simulink model "Mooventure2016_Rev5"  (Simulink 7.7)
settings: Solver=FixedStepDiscrete  StartTime=0.0  StopTime=10  RelTol=1e-3
PreLoadFcn:
  | try, eval([bdroot '_setup']); catch, eval('model_setup', ''); end
InitFcn:
  | try, eval([bdroot '_setup']); catch, eval('model_setup', ''); end
undefined symbols (not defined in the file): ECM, H1, motohawk_build_version, motohawk_trunc_name, motohawk_vardec_config_group, motohawk_vardec_path, xD
libraries: MotoHawk_lib x976, motohawk_control_primitives_lib x41, simulink x27, motohawk_annotations_lib x3
(part 12 of 16)

== system Mooventure2016_Rev5/Foreground/Control/Faults/Accesories/Blend Valves ==
  In1 : Inport
  Abs : Abs
  Abs1 : Abs
  Add1 : Sum  Inputs=+-
  Add2 : Sum  Inputs=+-
  Bus Selector1 : BusSelector  OutputSignals=Analog_Inputs.Coolant.Heater_Core_Blend_Position
  Bus Selector2 : BusSelector  OutputSignals=Analog_Inputs.Coolant.Radiator_Blend_Position
  Bus Selector3 : BusSelector  OutputSignals=Analog_Inputs.Coolant.Radiator_Blend_Position
  Bus Selector4 : BusSelector  OutputSignals=Analog_Inputs.Coolant.Radiator_Blend_Position
  Bus Selector5 : BusSelector  OutputSignals=Analog_Inputs.Coolant.Heater_Core_Blend_Position
  Bus Selector6 : BusSelector  OutputSignals=Analog_Inputs.Coolant.Heater_Core_Blend_Position
  Logical Operator : Logic  AllPortsSameDT=off  OutDataTypeStr=boolean
  Logical Operator1 : Logic  AllPortsSameDT=off  OutDataTypeStr=boolean
  Relational Operator{,4,6..7} (4 alike) : RelationalOperator  Operator=>  OutDataTypeStr=boolean
  Relational Operator1 : RelationalOperator  OutDataTypeStr=boolean
  Relational Operator2 : RelationalOperator  OutDataTypeStr=boolean
  Relational Operator3 : RelationalOperator  Operator=<  OutDataTypeStr=boolean
  Relational Operator5 : RelationalOperator  Operator=<  OutDataTypeStr=boolean
  Time Since Enabled (With Input)1 : motohawk_control_primitives_lib/Time Since Enabled (With Input)1  SystemSampleTime=-1  nam='TimeSinceRun1'  samp_time=-1  init=0  upperlim=16000
  Time Since Enabled (With Input)2 : motohawk_control_primitives_lib/Time Since Enabled (With Input)1  SystemSampleTime=-1  nam='TimeSinceRun2'  samp_time=-1  init=0  upperlim=16000
  Unit Delay : UnitDelay  SampleTime=-1
  Unit Delay1 : UnitDelay  SampleTime=-1
  motohawk_calibration : MotoHawk_lib/Calibration & Probing Blocks/motohawk_calibration  nam='Blend_Valve_A_No_Response_Fault'  val=100  storage=Calibration  show_more=off  name_source=Use Parameter  data_type=Inherit from 'Default Value'  read_level=1  write_level=1  ovr_cals=on  view_as=Number  enum_struct={'Disabled', 'Enabled'}  vector_style=Wide Row  use_help_units=off  help=''  units=''  use_header_enum=off  row_header_enum={}  col_header_enum={}  use_min_max=off  min_val=-inf  max_val=inf  use_precision=off  precision=''  gain=1  offset=0  exp=1  use_mototune_group=off  mototune_group=motohawk_vardec_path(gcb)
  motohawk_calibration1 : MotoHawk_lib/Calibration & Probing Blocks/motohawk_calibration  nam='Blend_Valve_Sensor_B_Intermittent_Fault'  val=4  storage=Calibration  show_more=off  name_source=Use Parameter  data_type=Inherit from 'Default Value'  read_level=1  write_level=1  ovr_cals=on  view_as=Number  enum_struct={'Disabled', 'Enabled'}  vector_style=Wide Row  use_help_units=off  help=''  units=''  use_header_enum=off  row_header_enum={}  col_header_enum={}  use_min_max=off  min_val=-inf  max_val=inf  use_precision=off  precision=''  gain=1  offset=0  exp=1  use_mototune_group=off  mototune_group=motohawk_vardec_path(gcb)
  motohawk_calibration2 : MotoHawk_lib/Calibration & Probing Blocks/motohawk_calibration  nam='Blend_Valve_Sensor_A_Intermittent_Fault'  val=4  storage=Calibration  show_more=off  name_source=Use Parameter  data_type=Inherit from 'Default Value'  read_level=1  write_level=1  ovr_cals=on  view_as=Number  enum_struct={'Disabled', 'Enabled'}  vector_style=Wide Row  use_help_units=off  help=''  units=''  use_header_enum=off  row_header_enum={}  col_header_enum={}  use_min_max=off  min_val=-inf  max_val=inf  use_precision=off  precision=''  gain=1  offset=0  exp=1  use_mototune_group=off  mototune_group=motohawk_vardec_path(gcb)
  motohawk_calibration3 : MotoHawk_lib/Calibration & Probing Blocks/motohawk_calibration  nam='Blend_Valve_Sensor_A_Low_Voltage_Fault'  val=5  storage=Calibration  show_more=off  name_source=Use Parameter  data_type=Inherit from 'Default Value'  read_level=1  write_level=1  ovr_cals=on  view_as=Number  enum_struct={'Disabled', 'Enabled'}  vector_style=Wide Row  use_help_units=off  help=''  units=''  use_header_enum=off  row_header_enum={}  col_header_enum={}  use_min_max=off  min_val=-inf  max_val=inf  use_precision=off  precision=''  gain=1  offset=0  exp=1  use_mototune_group=off  mototune_group=motohawk_vardec_path(gcb)
  motohawk_calibration4 : MotoHawk_lib/Calibration & Probing Blocks/motohawk_calibration  nam='Blend_Valve_Sensor_A_High_Voltage_Fault'  val=250  storage=Calibration  show_more=off  name_source=Use Parameter  data_type=Inherit from 'Default Value'  read_level=1  write_level=1  ovr_cals=on  view_as=Number  enum_struct={'Disabled', 'Enabled'}  vector_style=Wide Row  use_help_units=off  help=''  units=''  use_header_enum=off  row_header_enum={}  col_header_enum={}  use_min_max=off  min_val=-inf  max_val=inf  use_precision=off  precision=''  gain=1  offset=0  exp=1  use_mototune_group=off  mototune_group=motohawk_vardec_path(gcb)
  motohawk_calibration5 : MotoHawk_lib/Calibration & Probing Blocks/motohawk_calibration  nam='Blend_Valve_Sensor_B_Low_Voltage_Fault'  val=5  storage=Calibration  show_more=off  name_source=Use Parameter  data_type=Inherit from 'Default Value'  read_level=1  write_level=1  ovr_cals=on  view_as=Number  enum_struct={'Disabled', 'Enabled'}  vector_style=Wide Row  use_help_units=off  help=''  units=''  use_header_enum=off  row_header_enum={}  col_header_enum={}  use_min_max=off  min_val=-inf  max_val=inf  use_precision=off  precision=''  gain=1  offset=0  exp=1  use_mototune_group=off  mototune_group=motohawk_vardec_path(gcb)
  motohawk_calibration6 : MotoHawk_lib/Calibration & Probing Blocks/motohawk_calibration  nam='Blend_Valve_Sensor_B_High_Voltage_Fault'  val=250  storage=Calibration  show_more=off  name_source=Use Parameter  data_type=Inherit from 'Default Value'  read_level=1  write_level=1  ovr_cals=on  view_as=Number  enum_struct={'Disabled', 'Enabled'}  vector_style=Wide Row  use_help_units=off  help=''  units=''  use_header_enum=off  row_header_enum={}  col_header_enum={}  use_min_max=off  min_val=-inf  max_val=inf  use_precision=off  precision=''  gain=1  offset=0  exp=1  use_mototune_group=off  mototune_group=motohawk_vardec_path(gcb)
  motohawk_calibration7 : MotoHawk_lib/Calibration & Probing Blocks/motohawk_calibration  nam='Blend_Valve_B_No_Response_Fault'  val=100  storage=Calibration  show_more=off  name_source=Use Parameter  data_type=Inherit from 'Default Value'  read_level=1  write_level=1  ovr_cals=on  view_as=Number  enum_struct={'Disabled', 'Enabled'}  vector_style=Wide Row  use_help_units=off  help=''  units=''  use_header_enum=off  row_header_enum={}  col_header_enum={}  use_min_max=off  min_val=-inf  max_val=inf  use_precision=off  precision=''  gain=1  offset=0  exp=1  use_mototune_group=off  mototune_group=motohawk_vardec_path(gcb)
  motohawk_fault_def1 : MotoHawk_lib/Fault Management Blocks/motohawk_fault_def  nam='Blend_Valve_Sensor_B_Intermittent'  mode=Enabled  id=['B1B43']  x=9  y=10  input_suspected=on  indeterminate=off  increment_xy=on  downsample_count=1  ovr_cals=on  ovr_actions=on  show_actions=on  action1_name=''  action1_cond=(None)  action2_name=''  action2_cond=(None)  action3_name=''  action3_cond=(None)  action4_name=''  action4_cond=(None)
  motohawk_fault_def2 : MotoHawk_lib/Fault Management Blocks/motohawk_fault_def  nam='Blend_Valve_Sensor_B_Low_Voltage'  mode=Enabled  id=['B1B44']  x=9  y=10  input_suspected=on  indeterminate=off  increment_xy=on  downsample_count=1  ovr_cals=on  ovr_actions=on  show_actions=on  action1_name=''  action1_cond=(None)  action2_name=''  action2_cond=(None)  action3_name=''  action3_cond=(None)  action4_name=''  action4_cond=(None)
  motohawk_fault_def3 : MotoHawk_lib/Fault Management Blocks/motohawk_fault_def  nam='Blend_Valve_Sensor_A_Intermittent'  mode=Enabled  id=['B1B40']  x=9  y=10  input_suspected=on  indeterminate=off  increment_xy=on  downsample_count=1  ovr_cals=on  ovr_actions=on  show_actions=on  action1_name=''  action1_cond=(None)  action2_name=''  action2_cond=(None)  action3_name=''  action3_cond=(None)  action4_name=''  action4_cond=(None)
  motohawk_fault_def4 : MotoHawk_lib/Fault Management Blocks/motohawk_fault_def  nam='Blend_Valve_Sensor_A_Low_Voltage'  mode=Enabled  id=['B1B41']  x=9  y=10  input_suspected=on  indeterminate=off  increment_xy=on  downsample_count=1  ovr_cals=on  ovr_actions=on  show_actions=on  action1_name=''  action1_cond=(None)  action2_name=''  action2_cond=(None)  action3_name=''  action3_cond=(None)  action4_name=''  action4_cond=(None)
  motohawk_fault_def5 : MotoHawk_lib/Fault Management Blocks/motohawk_fault_def  nam='Blend_Valve_Sensor_A_High_Voltage'  mode=Enabled  id=['B1B42']  x=9  y=10  input_suspected=on  indeterminate=off  increment_xy=on  downsample_count=1  ovr_cals=on  ovr_actions=on  show_actions=on  action1_name=''  action1_cond=(None)  action2_name=''  action2_cond=(None)  action3_name=''  action3_cond=(None)  action4_name=''  action4_cond=(None)
  motohawk_fault_def6 : MotoHawk_lib/Fault Management Blocks/motohawk_fault_def  nam='Blend_Valve_Sensor_B_High_Voltage'  mode=Enabled  id=['B1B45']  x=9  y=10  input_suspected=on  indeterminate=off  increment_xy=on  downsample_count=1  ovr_cals=on  ovr_actions=on  show_actions=on  action1_name=''  action1_cond=(None)  action2_name=''  action2_cond=(None)  action3_name=''  action3_cond=(None)  action4_name=''  action4_cond=(None)
  motohawk_fault_def7 : MotoHawk_lib/Fault Management Blocks/motohawk_fault_def  nam='Blend_Valve_A_No_Response'  mode=Enabled  id=['B1B46']  x=9  y=10  input_suspected=on  indeterminate=off  increment_xy=on  downsample_count=1  ovr_cals=on  ovr_actions=on  show_actions=on  action1_name=''  action1_cond=(None)  action2_name=''  action2_cond=(None)  action3_name=''  action3_cond=(None)  action4_name=''  action4_cond=(None)
  motohawk_fault_def8 : MotoHawk_lib/Fault Management Blocks/motohawk_fault_def  nam='Blend_Valve_B_No_Response'  mode=Enabled  id=['B1B47']  x=9  y=10  input_suspected=on  indeterminate=off  increment_xy=on  downsample_count=1  ovr_cals=on  ovr_actions=on  show_actions=on  action1_name=''  action1_cond=(None)  action2_name=''  action2_cond=(None)  action3_name=''  action3_cond=(None)  action4_name=''  action4_cond=(None)
  wires:
  Bus Selector2/1 -> Add1/1, Unit Delay/1  "<Radiator_Blend_Position>"
  Unit Delay/1 -> Add1/2
  Add1/1 -> Abs/1
  Abs/1 -> Relational Operator2/1
  Relational Operator2/1 -> motohawk_fault_def3/1
  motohawk_calibration2/1 -> Relational Operator2/2
  motohawk_calibration3/1 -> Relational Operator3/2
  Relational Operator3/1 -> motohawk_fault_def4/1
  Bus Selector3/1 -> Relational Operator3/1  "<Radiator_Blend_Position>"
  motohawk_calibration4/1 -> Relational Operator4/2
  Relational Operator4/1 -> motohawk_fault_def5/1
  Bus Selector4/1 -> Relational Operator4/1  "<Radiator_Blend_Position>"
  In1/1 -> Bus Selector2/1, Bus Selector3/1, Bus Selector4/1, Bus Selector1/1, Bus Selector5/1, Bus Selector6/1
  Bus Selector1/1 -> Add2/1, Unit Delay1/1  "<Heater_Core_Blend_Position>"
  Unit Delay1/1 -> Add2/2
  Add2/1 -> Abs1/1
  Abs1/1 -> Relational Operator1/1
  Relational Operator1/1 -> motohawk_fault_def1/1
  motohawk_calibration1/1 -> Relational Operator1/2
  motohawk_calibration5/1 -> Relational Operator5/2
  Relational Operator5/1 -> motohawk_fault_def2/1
  Bus Selector5/1 -> Relational Operator5/1  "<Heater_Core_Blend_Position>"
  motohawk_calibration6/1 -> Relational Operator6/2
  Relational Operator6/1 -> motohawk_fault_def6/1
  Bus Selector6/1 -> Relational Operator6/1  "<Heater_Core_Blend_Position>"
  [RadiatorMotor] -> Time Since Enabled (With Input)1/1, Logical Operator/2
  [HeaterMotor] -> Time Since Enabled (With Input)2/1, Logical Operator1/2
  motohawk_calibration/1 -> Relational Operator/2
  Time Since Enabled (With Input)1/1 -> Relational Operator/1
  Time Since Enabled (With Input)2/1 -> Relational Operator7/1
  motohawk_calibration7/1 -> Relational Operator7/2
  Relational Operator/1 -> Logical Operator/1
  Relational Operator7/1 -> Logical Operator1/1
  Logical Operator/1 -> motohawk_fault_def7/1
  Logical Operator1/1 -> motohawk_fault_def8/1

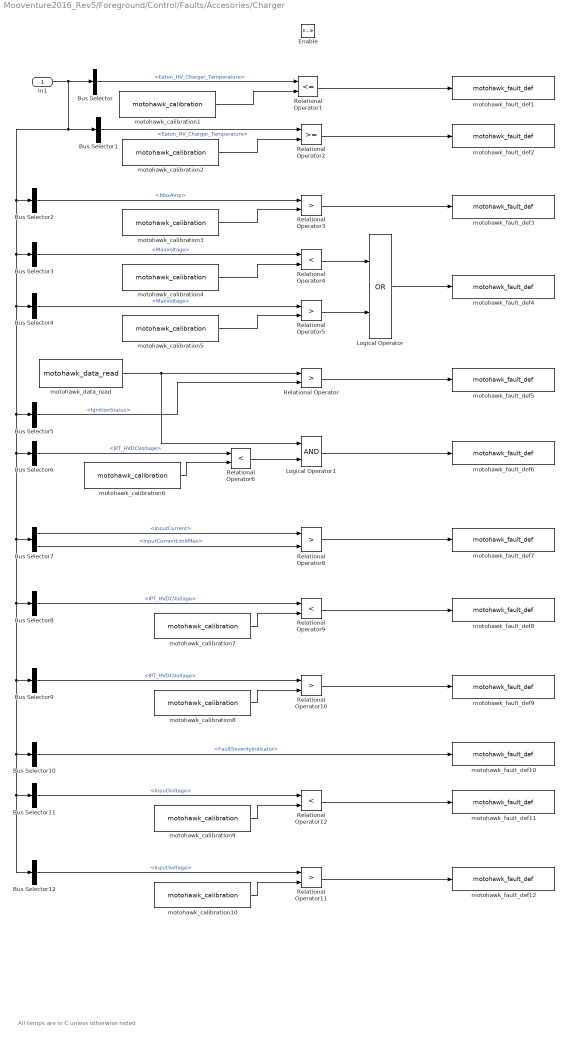
== system Mooventure2016_Rev5/Foreground/Control/Faults/Accesories/Charger ==
  note: All temps are in C unless otherwise noted
  In1 : Inport
  Enable : EnablePort
  Bus Selector : BusSelector  OutputSignals=Eaton_Charger.Eaton_Charger.Eaton_HV_Charger_Temperature
  Bus Selector1 : BusSelector  OutputSignals=Eaton_Charger.Eaton_Charger.Eaton_HV_Charger_Temperature
  Bus Selector10 : BusSelector  OutputSignals=Eaton_Charger.Eaton_Charger.FaultSeverityIndicator
  Bus Selector11 : BusSelector  OutputSignals=Eaton_Charger.Eaton_Charger.InputVoltage
  Bus Selector12 : BusSelector  OutputSignals=Eaton_Charger.Eaton_Charger.InputVoltage
  Bus Selector2 : BusSelector  OutputSignals=ChargerParam.MaxAmp
  Bus Selector3 : BusSelector  OutputSignals=ChargerParam.MaxVoltage
  Bus Selector4 : BusSelector  OutputSignals=ChargerParam.MaxVoltage
  Bus Selector5 : BusSelector  OutputSignals=Eaton_Charger.Eaton_Charger.IgnitionStatus
  Bus Selector6 : BusSelector  OutputSignals=IPT.ID 278 IPT Status 1.IPT_HVDCVoltage
  Bus Selector7 : BusSelector  OutputSignals=Eaton_Charger.Eaton_Charger.InputCurrent,Eaton_Charger.Eaton_Charger.InputCurrentLimitMax
  Bus Selector8 : BusSelector  OutputSignals=IPT.ID 278 IPT Status 1.IPT_HVDCVoltage
  Bus Selector9 : BusSelector  OutputSignals=IPT.ID 278 IPT Status 1.IPT_HVDCVoltage
  Logical Operator : Logic  Operator=OR  AllPortsSameDT=off  OutDataTypeStr=boolean
  Logical Operator1 : Logic  AllPortsSameDT=off  OutDataTypeStr=boolean
  Relational Operator{,3,5,8,10..11} (6 alike) : RelationalOperator  Operator=>  OutDataTypeStr=boolean
  Relational Operator1 : RelationalOperator  Operator=<=  OutDataTypeStr=boolean
  Relational Operator{4,6,9,12} (4 alike) : RelationalOperator  Operator=<  OutDataTypeStr=boolean
  Relational Operator2 : RelationalOperator  OutDataTypeStr=boolean
  motohawk_calibration1 : MotoHawk_lib/Calibration & Probing Blocks/motohawk_calibration  nam='Charger_Derated_Under_Temperature_Fault'  val=-30  storage=Calibration  show_more=off  name_source=Use Parameter  data_type=Inherit from 'Default Value'  read_level=1  write_level=1  ovr_cals=on  view_as=Number  enum_struct={'Disabled', 'Enabled'}  vector_style=Wide Row  use_help_units=off  help=''  units=''  use_header_enum=off  row_header_enum={}  col_header_enum={}  use_min_max=off  min_val=-inf  max_val=inf  use_precision=off  precision=''  gain=1  offset=0  exp=1  use_mototune_group=off  mototune_group=motohawk_vardec_path(gcb)
  motohawk_calibration10 : MotoHawk_lib/Calibration & Probing Blocks/motohawk_calibration  nam='Charger_Line_Votlage_Too_High_Fault'  val=300  storage=Calibration  show_more=off  name_source=Use Parameter  data_type=Inherit from 'Default Value'  read_level=1  write_level=1  ovr_cals=on  view_as=Number  enum_struct={'Disabled', 'Enabled'}  vector_style=Wide Row  use_help_units=off  help=''  units=''  use_header_enum=off  row_header_enum={}  col_header_enum={}  use_min_max=off  min_val=-inf  max_val=inf  use_precision=off  precision=''  gain=1  offset=0  exp=1  use_mototune_group=off  mototune_group=motohawk_vardec_path(gcb)
  motohawk_calibration2 : MotoHawk_lib/Calibration & Probing Blocks/motohawk_calibration  nam='Charger_Derated_Over_Temperature_Fault'  val=60  storage=Calibration  show_more=off  name_source=Use Parameter  data_type=Inherit from 'Default Value'  read_level=1  write_level=1  ovr_cals=on  view_as=Number  enum_struct={'Disabled', 'Enabled'}  vector_style=Wide Row  use_help_units=off  help=''  units=''  use_header_enum=off  row_header_enum={}  col_header_enum={}  use_min_max=off  min_val=-inf  max_val=inf  use_precision=off  precision=''  gain=1  offset=0  exp=1  use_mototune_group=off  mototune_group=motohawk_vardec_path(gcb)
  motohawk_calibration3 : MotoHawk_lib/Calibration & Probing Blocks/motohawk_calibration  nam='Charger_Requested_Current_Too_High_Fault'  val=16  storage=Calibration  show_more=off  name_source=Use Parameter  data_type=Inherit from 'Default Value'  read_level=1  write_level=1  ovr_cals=on  view_as=Number  enum_struct={'Disabled', 'Enabled'}  vector_style=Wide Row  use_help_units=off  help=''  units=''  use_header_enum=off  row_header_enum={}  col_header_enum={}  use_min_max=off  min_val=-inf  max_val=inf  use_precision=off  precision=''  gain=1  offset=0  exp=1  use_mototune_group=off  mototune_group=motohawk_vardec_path(gcb)
  motohawk_calibration4 : MotoHawk_lib/Calibration & Probing Blocks/motohawk_calibration  nam='Charger_Requested_Voltage_Out_of_Bounds_Fault_Lower'  val=298  storage=Calibration  show_more=off  name_source=Use Parameter  data_type=Inherit from 'Default Value'  read_level=1  write_level=1  ovr_cals=on  view_as=Number  enum_struct={'Disabled', 'Enabled'}  vector_style=Wide Row  use_help_units=off  help=''  units=''  use_header_enum=off  row_header_enum={}  col_header_enum={}  use_min_max=off  min_val=-inf  max_val=inf  use_precision=off  precision=''  gain=1  offset=0  exp=1  use_mototune_group=off  mototune_group=motohawk_vardec_path(gcb)
  motohawk_calibration5 : MotoHawk_lib/Calibration & Probing Blocks/motohawk_calibration  nam='Charger_Requested_Voltage_Out_of_Bounds_Fault_Upper'  val=428  storage=Calibration  show_more=off  name_source=Use Parameter  data_type=Inherit from 'Default Value'  read_level=1  write_level=1  ovr_cals=on  view_as=Number  enum_struct={'Disabled', 'Enabled'}  vector_style=Wide Row  use_help_units=off  help=''  units=''  use_header_enum=off  row_header_enum={}  col_header_enum={}  use_min_max=off  min_val=-inf  max_val=inf  use_precision=off  precision=''  gain=1  offset=0  exp=1  use_mototune_group=off  mototune_group=motohawk_vardec_path(gcb)
  motohawk_calibration6 : MotoHawk_lib/Calibration & Probing Blocks/motohawk_calibration  nam='Charger_Requested_But_No_High_Voltage_Fault'  val=50  storage=Calibration  show_more=off  name_source=Use Parameter  data_type=Inherit from 'Default Value'  read_level=1  write_level=1  ovr_cals=on  view_as=Number  enum_struct={'Disabled', 'Enabled'}  vector_style=Wide Row  use_help_units=off  help=''  units=''  use_header_enum=off  row_header_enum={}  col_header_enum={}  use_min_max=off  min_val=-inf  max_val=inf  use_precision=off  precision=''  gain=1  offset=0  exp=1  use_mototune_group=off  mototune_group=motohawk_vardec_path(gcb)
  motohawk_calibration7 : MotoHawk_lib/Calibration & Probing Blocks/motohawk_calibration  nam='Battery_Voltage_Too_Low_Fault'  val=200  storage=Calibration  show_more=off  name_source=Use Parameter  data_type=Inherit from 'Default Value'  read_level=1  write_level=1  ovr_cals=on  view_as=Number  enum_struct={'Disabled', 'Enabled'}  vector_style=Wide Row  use_help_units=off  help=''  units=''  use_header_enum=off  row_header_enum={}  col_header_enum={}  use_min_max=off  min_val=-inf  max_val=inf  use_precision=off  precision=''  gain=1  offset=0  exp=1  use_mototune_group=off  mototune_group=motohawk_vardec_path(gcb)
  motohawk_calibration8 : MotoHawk_lib/Calibration & Probing Blocks/motohawk_calibration  nam='Battery_Voltage_Too_High_Fault'  val=400  storage=Calibration  show_more=off  name_source=Use Parameter  data_type=Inherit from 'Default Value'  read_level=1  write_level=1  ovr_cals=on  view_as=Number  enum_struct={'Disabled', 'Enabled'}  vector_style=Wide Row  use_help_units=off  help=''  units=''  use_header_enum=off  row_header_enum={}  col_header_enum={}  use_min_max=off  min_val=-inf  max_val=inf  use_precision=off  precision=''  gain=1  offset=0  exp=1  use_mototune_group=off  mototune_group=motohawk_vardec_path(gcb)
  motohawk_calibration9 : MotoHawk_lib/Calibration & Probing Blocks/motohawk_calibration  nam='Charger_Line_Voltage_Too_Low_Fault'  val=100  storage=Calibration  show_more=off  name_source=Use Parameter  data_type=Inherit from 'Default Value'  read_level=1  write_level=1  ovr_cals=on  view_as=Number  enum_struct={'Disabled', 'Enabled'}  vector_style=Wide Row  use_help_units=off  help=''  units=''  use_header_enum=off  row_header_enum={}  col_header_enum={}  use_min_max=off  min_val=-inf  max_val=inf  use_precision=off  precision=''  gain=1  offset=0  exp=1  use_mototune_group=off  mototune_group=motohawk_vardec_path(gcb)
  motohawk_data_read : MotoHawk_lib/Data Storage Blocks/motohawk_data_read  source=Lookup By Name  structure=Scalar  operation=Read scalar from location by index  sz_vec=4  sz_row=2  sz_col=3  typ=boolean  nam='ChargeEnable'  checkNull=on  struct_inst_name='MyData'  struct_nam='MyStruct'
  motohawk_fault_def1 : MotoHawk_lib/Fault Management Blocks/motohawk_fault_def  nam='Charger_Derated_Under_Temperature'  mode=Enabled  id=['B1A10']  x=9  y=10  input_suspected=on  indeterminate=off  increment_xy=on  downsample_count=1  ovr_cals=on  ovr_actions=on  show_actions=on  action1_name='Temperature_Flash'  action1_cond=(None)  action2_name=''  action2_cond=(None)  action3_name=''  action3_cond=(None)  action4_name=''  action4_cond=(None)
  motohawk_fault_def10 : MotoHawk_lib/Fault Management Blocks/motohawk_fault_def  nam='Charger_Internal_Fault'  mode=Enabled  id=['B1A32']  x=9  y=10  input_suspected=on  indeterminate=off  increment_xy=on  downsample_count=1  ovr_cals=on  ovr_actions=on  show_actions=on  action1_name='HV_Light'  action1_cond=Active  action2_name=''  action2_cond=(None)  action3_name=''  action3_cond=(None)  action4_name=''  action4_cond=(None)
  motohawk_fault_def11 : MotoHawk_lib/Fault Management Blocks/motohawk_fault_def  nam='Charger_Line_Voltage_Too_Low'  mode=Enabled  id=['B1A33']  x=9  y=10  input_suspected=on  indeterminate=off  increment_xy=on  downsample_count=1  ovr_cals=on  ovr_actions=on  show_actions=on  action1_name='Wrench_Light'  action1_cond=Active  action2_name=''  action2_cond=(None)  action3_name=''  action3_cond=(None)  action4_name=''  action4_cond=(None)
  motohawk_fault_def12 : MotoHawk_lib/Fault Management Blocks/motohawk_fault_def  nam='Charger_Line_Votlage_Too_High'  mode=Enabled  id=['B1A34']  x=9  y=10  input_suspected=on  indeterminate=off  increment_xy=on  downsample_count=1  ovr_cals=on  ovr_actions=on  show_actions=on  action1_name='Wrench_Light'  action1_cond=Active  action2_name=''  action2_cond=(None)  action3_name=''  action3_cond=(None)  action4_name=''  action4_cond=(None)
  motohawk_fault_def2 : MotoHawk_lib/Fault Management Blocks/motohawk_fault_def  nam='Charger_Derated_Over_Temperature'  mode=Enabled  id=['B1A11']  x=9  y=10  input_suspected=on  indeterminate=off  increment_xy=on  downsample_count=1  ovr_cals=on  ovr_actions=on  show_actions=on  action1_name='Temperature_Solid'  action1_cond=Active  action2_name='Cooling_Max'  action2_cond=(None)  action3_name=''  action3_cond=(None)  action4_name=''  action4_cond=(None)
  motohawk_fault_def3 : MotoHawk_lib/Fault Management Blocks/motohawk_fault_def  nam='Charger_Requested_Current_Too_High'  mode=Enabled  id=['B1A20']  x=9  y=10  input_suspected=on  indeterminate=off  increment_xy=on  downsample_count=1  ovr_cals=on  ovr_actions=on  show_actions=on  action1_name='HV_Light'  action1_cond=Active  action2_name=''  action2_cond=(None)  action3_name=''  action3_cond=(None)  action4_name=''  action4_cond=(None)
  motohawk_fault_def4 : MotoHawk_lib/Fault Management Blocks/motohawk_fault_def  nam='Charger_Requested_Voltage_Out_of_Bounds'  mode=Enabled  id=['B1A21']  x=9  y=10  input_suspected=on  indeterminate=off  increment_xy=on  downsample_count=1  ovr_cals=on  ovr_actions=on  show_actions=on  action1_name='HV_Light'  action1_cond=Active  action2_name=''  action2_cond=(None)  action3_name=''  action3_cond=(None)  action4_name=''  action4_cond=(None)
  motohawk_fault_def5 : MotoHawk_lib/Fault Management Blocks/motohawk_fault_def  nam='Charger_Requested_But_No_Key_Singal'  mode=Enabled  id=['B1A22']  x=9  y=10  input_suspected=on  indeterminate=off  increment_xy=on  downsample_count=1  ovr_cals=on  ovr_actions=on  show_actions=on  action1_name='Wrench_Light'  action1_cond=Active  action2_name=''  action2_cond=(None)  action3_name=''  action3_cond=(None)  action4_name=''  action4_cond=(None)
  motohawk_fault_def6 : MotoHawk_lib/Fault Management Blocks/motohawk_fault_def  nam='Charger_Requested_But_No_High_Voltage'  mode=Enabled  id=['B1A23']  x=9  y=10  input_suspected=on  indeterminate=off  increment_xy=on  downsample_count=1  ovr_cals=on  ovr_actions=on  show_actions=on  action1_name='HV_Light'  action1_cond=Active  action2_name=''  action2_cond=(None)  action3_name=''  action3_cond=(None)  action4_name=''  action4_cond=(None)
  motohawk_fault_def7 : MotoHawk_lib/Fault Management Blocks/motohawk_fault_def  nam='Charger_Amperage_Draw_Greater_Then_Supply'  mode=Enabled  id=['B1A24']  x=9  y=10  input_suspected=on  indeterminate=off  increment_xy=on  downsample_count=1  ovr_cals=on  ovr_actions=on  show_actions=on  action1_name='HV_Light'  action1_cond=Active  action2_name=''  action2_cond=(None)  action3_name=''  action3_cond=(None)  action4_name=''  action4_cond=(None)
  motohawk_fault_def8 : MotoHawk_lib/Fault Management Blocks/motohawk_fault_def  nam='Battery_Voltage_Too_Low'  mode=Enabled  id=['B1A30']  x=9  y=10  input_suspected=on  indeterminate=off  increment_xy=on  downsample_count=1  ovr_cals=on  ovr_actions=on  show_actions=on  action1_name='HV_Light'  action1_cond=Active  action2_name=''  action2_cond=(None)  action3_name=''  action3_cond=(None)  action4_name=''  action4_cond=(None)
  motohawk_fault_def9 : MotoHawk_lib/Fault Management Blocks/motohawk_fault_def  nam='Battery_Voltage_Too_High'  mode=Enabled  id=['B1A31']  x=9  y=10  input_suspected=on  indeterminate=off  increment_xy=on  downsample_count=1  ovr_cals=on  ovr_actions=on  show_actions=on  action1_name='HV_Light'  action1_cond=Active  action2_name=''  action2_cond=(None)  action3_name=''  action3_cond=(None)  action4_name=''  action4_cond=(None)
  wires:
  In1/1 -> Bus Selector/1, Bus Selector1/1, Bus Selector2/1, Bus Selector5/1, Bus Selector6/1, Bus Selector7/1, Bus Selector8/1, Bus Selector9/1, Bus Selector10/1, Bus Selector11/1, Bus Selector12/1, Bus Selector4/1, Bus Selector3/1
  motohawk_calibration1/1 -> Relational Operator1/2
  Relational Operator1/1 -> motohawk_fault_def1/1
  Bus Selector/1 -> Relational Operator1/1  "<Eaton_HV_Charger_Temperature>"
  motohawk_calibration2/1 -> Relational Operator2/2
  Relational Operator2/1 -> motohawk_fault_def2/1
  Bus Selector1/1 -> Relational Operator2/1  "<Eaton_HV_Charger_Temperature>"
  motohawk_calibration3/1 -> Relational Operator3/2
  Relational Operator3/1 -> motohawk_fault_def3/1
  motohawk_calibration4/1 -> Relational Operator4/2
  motohawk_calibration5/1 -> Relational Operator5/2
  Relational Operator4/1 -> Logical Operator/1
  Relational Operator5/1 -> Logical Operator/2
  Logical Operator/1 -> motohawk_fault_def4/1
  Bus Selector5/1 -> Relational Operator/2  "<IgnitionStatus>"
  Relational Operator/1 -> motohawk_fault_def5/1
  motohawk_calibration6/1 -> Relational Operator6/2
  Bus Selector6/1 -> Relational Operator6/1  "<IPT_HVDCVoltage>"
  Relational Operator6/1 -> Logical Operator1/2
  Logical Operator1/1 -> motohawk_fault_def6/1
  Bus Selector7/1 -> Relational Operator8/1  "<InputCurrent>"
  Bus Selector7/2 -> Relational Operator8/2  "<InputCurrentLimitMax>"
  Relational Operator8/1 -> motohawk_fault_def7/1
  motohawk_calibration7/1 -> Relational Operator9/2
  Bus Selector8/1 -> Relational Operator9/1  "<IPT_HVDCVoltage>"
  Relational Operator9/1 -> motohawk_fault_def8/1
  motohawk_calibration8/1 -> Relational Operator10/2
  Bus Selector9/1 -> Relational Operator10/1  "<IPT_HVDCVoltage>"
  Relational Operator10/1 -> motohawk_fault_def9/1
  Bus Selector10/1 -> motohawk_fault_def10/1  "<FaultSeverityIndicator>"
  motohawk_calibration9/1 -> Relational Operator12/2
  Bus Selector11/1 -> Relational Operator12/1  "<InputVoltage>"
  Relational Operator12/1 -> motohawk_fault_def11/1
  motohawk_calibration10/1 -> Relational Operator11/2
  Bus Selector12/1 -> Relational Operator11/1  "<InputVoltage>"
  Relational Operator11/1 -> motohawk_fault_def12/1
  Bus Selector2/1 -> Relational Operator3/1  "<MaxAmp>"
  Bus Selector3/1 -> Relational Operator4/1  "<MaxVoltage>"
  Bus Selector4/1 -> Relational Operator5/1  "<MaxVoltage>"
  motohawk_data_read/1 -> Relational Operator/1, Logical Operator1/1

== system Mooventure2016_Rev5/Foreground/Control/Faults/Accesories/DC-DC Converter ==
  In1 : Inport
  Bus Selector : BusSelector  OutputSignals=Analog_Inputs.DCDC
  Relational Operator1 : RelationalOperator  Operator=<  OutDataTypeStr=boolean
  motohawk_calibration1 : MotoHawk_lib/Calibration & Probing Blocks/motohawk_calibration  nam='DCDC_Converter_Not_Running_Fault'  val=200  storage=Calibration  show_more=off  name_source=Use Parameter  data_type=Inherit from 'Default Value'  read_level=1  write_level=1  ovr_cals=on  view_as=Number  enum_struct={'Disabled', 'Enabled'}  vector_style=Wide Row  use_help_units=off  help=''  units=''  use_header_enum=off  row_header_enum={}  col_header_enum={}  use_min_max=off  min_val=-inf  max_val=inf  use_precision=off  precision=''  gain=1  offset=0  exp=1  use_mototune_group=off  mototune_group=motohawk_vardec_path(gcb)
  motohawk_fault_def1 : MotoHawk_lib/Fault Management Blocks/motohawk_fault_def  nam='DCDC_Converter_Not_Running'  mode=Disabled  id=['B1B11']  x=9  y=10  input_suspected=on  indeterminate=off  increment_xy=on  downsample_count=1  ovr_cals=on  ovr_actions=on  show_actions=on  action1_name='Batt_Light'  action1_cond=Active  action2_name=''  action2_cond=(None)  action3_name=''  action3_cond=(None)  action4_name=''  action4_cond=(None)
  wires:
  motohawk_calibration1/1 -> Relational Operator1/2
  Relational Operator1/1 -> motohawk_fault_def1/1
  Bus Selector/1 -> Relational Operator1/1  "<DCDC>"
  In1/1 -> Bus Selector/1

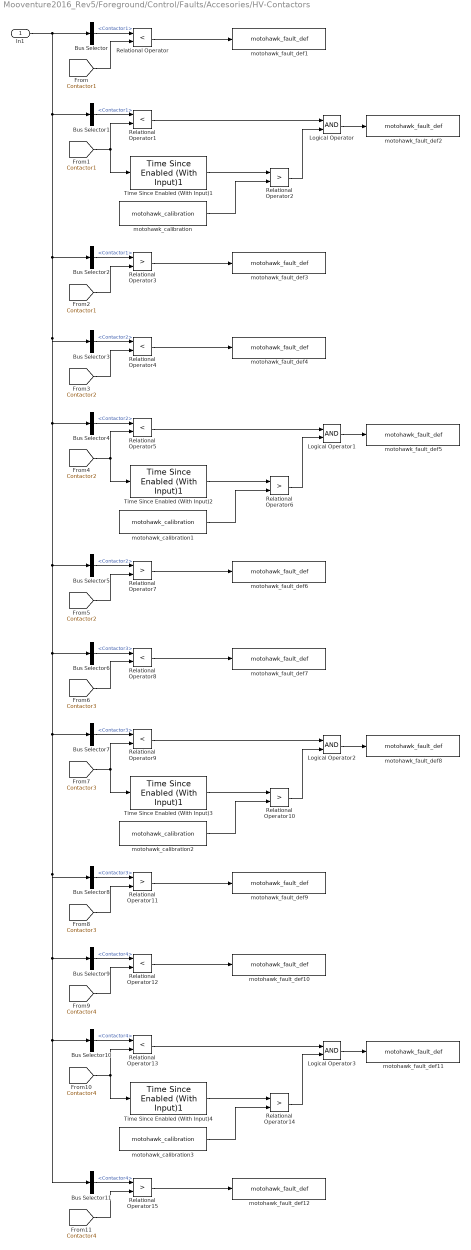
== system Mooventure2016_Rev5/Foreground/Control/Faults/Accesories/HV-Contactors ==
  In1 : Inport
  Bus Selector : BusSelector  OutputSignals=Analog_Inputs.Contactors.Contactor1
  Bus Selector1 : BusSelector  OutputSignals=Analog_Inputs.Contactors.Contactor1
  Bus Selector10 : BusSelector  OutputSignals=Analog_Inputs.Contactors.Contactor4
  Bus Selector11 : BusSelector  OutputSignals=Analog_Inputs.Contactors.Contactor4
  Bus Selector2 : BusSelector  OutputSignals=Analog_Inputs.Contactors.Contactor1
  Bus Selector3 : BusSelector  OutputSignals=Analog_Inputs.Contactors.Contactor2
  Bus Selector4 : BusSelector  OutputSignals=Analog_Inputs.Contactors.Contactor2
  Bus Selector5 : BusSelector  OutputSignals=Analog_Inputs.Contactors.Contactor2
  Bus Selector6 : BusSelector  OutputSignals=Analog_Inputs.Contactors.Contactor3
  Bus Selector7 : BusSelector  OutputSignals=Analog_Inputs.Contactors.Contactor3
  Bus Selector8 : BusSelector  OutputSignals=Analog_Inputs.Contactors.Contactor3
  Bus Selector9 : BusSelector  OutputSignals=Analog_Inputs.Contactors.Contactor4
  Logical Operator{,1..3} (4 alike) : Logic  AllPortsSameDT=off  OutDataTypeStr=boolean
  Relational Operator{,1,4..5,8..9,12..13} (8 alike) : RelationalOperator  Operator=<  OutDataTypeStr=boolean
  Relational Operator{2..3,6..7,10..11,14..15} (8 alike) : RelationalOperator  Operator=>  OutDataTypeStr=boolean
  Time Since Enabled (With Input)1 : motohawk_control_primitives_lib/Time Since Enabled (With Input)1  SystemSampleTime=-1  nam='ContactorOne'  samp_time=-1  init=0  upperlim=16000
  Time Since Enabled (With Input)2 : motohawk_control_primitives_lib/Time Since Enabled (With Input)1  SystemSampleTime=-1  nam='ContactorTwo'  samp_time=-1  init=0  upperlim=16000
  Time Since Enabled (With Input)3 : motohawk_control_primitives_lib/Time Since Enabled (With Input)1  SystemSampleTime=-1  nam='ContactorThree'  samp_time=-1  init=0  upperlim=16000
  Time Since Enabled (With Input)4 : motohawk_control_primitives_lib/Time Since Enabled (With Input)1  SystemSampleTime=-1  nam='ContactorFour'  samp_time=-1  init=0  upperlim=16000
  motohawk_calibration : MotoHawk_lib/Calibration & Probing Blocks/motohawk_calibration  nam='Contactor1_Unexpected_Open_Fault'  val=2  storage=Calibration  show_more=off  name_source=Use Parameter  data_type=Inherit from 'Default Value'  read_level=1  write_level=1  ovr_cals=on  view_as=Number  enum_struct={'Disabled', 'Enabled'}  vector_style=Wide Row  use_help_units=off  help=''  units=''  use_header_enum=off  row_header_enum={}  col_header_enum={}  use_min_max=off  min_val=-inf  max_val=inf  use_precision=off  precision=''  gain=1  offset=0  exp=1  use_mototune_group=off  mototune_group=motohawk_vardec_path(gcb)
  motohawk_calibration1 : MotoHawk_lib/Calibration & Probing Blocks/motohawk_calibration  nam='Contactor2_Unexpected_Open_Fault'  val=2  storage=Calibration  show_more=off  name_source=Use Parameter  data_type=Inherit from 'Default Value'  read_level=1  write_level=1  ovr_cals=on  view_as=Number  enum_struct={'Disabled', 'Enabled'}  vector_style=Wide Row  use_help_units=off  help=''  units=''  use_header_enum=off  row_header_enum={}  col_header_enum={}  use_min_max=off  min_val=-inf  max_val=inf  use_precision=off  precision=''  gain=1  offset=0  exp=1  use_mototune_group=off  mototune_group=motohawk_vardec_path(gcb)
  motohawk_calibration2 : MotoHawk_lib/Calibration & Probing Blocks/motohawk_calibration  nam='Contactor3_Unexpected_Open_Fault'  val=2  storage=Calibration  show_more=off  name_source=Use Parameter  data_type=Inherit from 'Default Value'  read_level=1  write_level=1  ovr_cals=on  view_as=Number  enum_struct={'Disabled', 'Enabled'}  vector_style=Wide Row  use_help_units=off  help=''  units=''  use_header_enum=off  row_header_enum={}  col_header_enum={}  use_min_max=off  min_val=-inf  max_val=inf  use_precision=off  precision=''  gain=1  offset=0  exp=1  use_mototune_group=off  mototune_group=motohawk_vardec_path(gcb)
  motohawk_calibration3 : MotoHawk_lib/Calibration & Probing Blocks/motohawk_calibration  nam='Contactor4_Unexpected_Open_Fault'  val=2  storage=Calibration  show_more=off  name_source=Use Parameter  data_type=Inherit from 'Default Value'  read_level=1  write_level=1  ovr_cals=on  view_as=Number  enum_struct={'Disabled', 'Enabled'}  vector_style=Wide Row  use_help_units=off  help=''  units=''  use_header_enum=off  row_header_enum={}  col_header_enum={}  use_min_max=off  min_val=-inf  max_val=inf  use_precision=off  precision=''  gain=1  offset=0  exp=1  use_mototune_group=off  mototune_group=motohawk_vardec_path(gcb)
  motohawk_fault_def1 : MotoHawk_lib/Fault Management Blocks/motohawk_fault_def  nam='Contactor_1_Failure_To_Close'  mode=Disabled  id=['B1B50']  x=1500  y=2000  input_suspected=on  indeterminate=off  increment_xy=on  downsample_count=1  ovr_cals=on  ovr_actions=on  show_actions=on  action1_name=''  action1_cond=(None)  action2_name=''  action2_cond=(None)  action3_name=''  action3_cond=(None)  action4_name=''  action4_cond=(None)
  motohawk_fault_def10 : MotoHawk_lib/Fault Management Blocks/motohawk_fault_def  nam='Contactor_4_Failure_To_Close'  mode=Disabled  id=['B1B59']  x=1500  y=2000  input_suspected=on  indeterminate=off  increment_xy=on  downsample_count=1  ovr_cals=on  ovr_actions=on  show_actions=on  action1_name=''  action1_cond=(None)  action2_name=''  action2_cond=(None)  action3_name=''  action3_cond=(None)  action4_name=''  action4_cond=(None)
  motohawk_fault_def11 : MotoHawk_lib/Fault Management Blocks/motohawk_fault_def  nam='Contactor_4_Unexpected_Open'  mode=Disabled  id=['B1B5A']  x=1500  y=2000  input_suspected=on  indeterminate=off  increment_xy=on  downsample_count=1  ovr_cals=on  ovr_actions=on  show_actions=on  action1_name=''  action1_cond=(None)  action2_name=''  action2_cond=(None)  action3_name=''  action3_cond=(None)  action4_name=''  action4_cond=(None)
  motohawk_fault_def12 : MotoHawk_lib/Fault Management Blocks/motohawk_fault_def  nam='Contactor_4_Fused'  mode=Disabled  id=['B1B5B']  x=9  y=10  input_suspected=on  indeterminate=off  increment_xy=on  downsample_count=1  ovr_cals=on  ovr_actions=on  show_actions=on  action1_name=''  action1_cond=(None)  action2_name=''  action2_cond=(None)  action3_name=''  action3_cond=(None)  action4_name=''  action4_cond=(None)
  motohawk_fault_def2 : MotoHawk_lib/Fault Management Blocks/motohawk_fault_def  nam='Contactor_1_Unexpected_Open'  mode=Disabled  id=['B1B51']  x=1500  y=2000  input_suspected=on  indeterminate=off  increment_xy=on  downsample_count=1  ovr_cals=on  ovr_actions=on  show_actions=on  action1_name=''  action1_cond=(None)  action2_name=''  action2_cond=(None)  action3_name=''  action3_cond=(None)  action4_name=''  action4_cond=(None)
  motohawk_fault_def3 : MotoHawk_lib/Fault Management Blocks/motohawk_fault_def  nam='Contactor_1_Fused'  mode=Disabled  id=['B1B52']  x=9  y=10  input_suspected=on  indeterminate=off  increment_xy=on  downsample_count=1  ovr_cals=on  ovr_actions=on  show_actions=on  action1_name=''  action1_cond=(None)  action2_name=''  action2_cond=(None)  action3_name=''  action3_cond=(None)  action4_name=''  action4_cond=(None)
  motohawk_fault_def4 : MotoHawk_lib/Fault Management Blocks/motohawk_fault_def  nam='Contactor_2_Failure_To_Close'  mode=Disabled  id=['B1B53']  x=1500  y=2000  input_suspected=on  indeterminate=off  increment_xy=on  downsample_count=1  ovr_cals=on  ovr_actions=on  show_actions=on  action1_name=''  action1_cond=(None)  action2_name=''  action2_cond=(None)  action3_name=''  action3_cond=(None)  action4_name=''  action4_cond=(None)
  motohawk_fault_def5 : MotoHawk_lib/Fault Management Blocks/motohawk_fault_def  nam='Contactor_2_Unexpected_Open'  mode=Disabled  id=['B1B54']  x=1500  y=2000  input_suspected=on  indeterminate=off  increment_xy=on  downsample_count=1  ovr_cals=on  ovr_actions=on  show_actions=on  action1_name=''  action1_cond=(None)  action2_name=''  action2_cond=(None)  action3_name=''  action3_cond=(None)  action4_name=''  action4_cond=(None)
  motohawk_fault_def6 : MotoHawk_lib/Fault Management Blocks/motohawk_fault_def  nam='Contactor_2_Fused'  mode=Disabled  id=['B1B55']  x=9  y=10  input_suspected=on  indeterminate=off  increment_xy=on  downsample_count=1  ovr_cals=on  ovr_actions=on  show_actions=on  action1_name=''  action1_cond=(None)  action2_name=''  action2_cond=(None)  action3_name=''  action3_cond=(None)  action4_name=''  action4_cond=(None)
  motohawk_fault_def7 : MotoHawk_lib/Fault Management Blocks/motohawk_fault_def  nam='Contactor_3_Failure_To_Close'  mode=Disabled  id=['B1B56']  x=1500  y=2000  input_suspected=on  indeterminate=off  increment_xy=on  downsample_count=1  ovr_cals=on  ovr_actions=on  show_actions=on  action1_name=''  action1_cond=(None)  action2_name=''  action2_cond=(None)  action3_name=''  action3_cond=(None)  action4_name=''  action4_cond=(None)
  motohawk_fault_def8 : MotoHawk_lib/Fault Management Blocks/motohawk_fault_def  nam='Contactor_3_Unexpected_Open'  mode=Disabled  id=['B1B57']  x=1500  y=2000  input_suspected=on  indeterminate=off  increment_xy=on  downsample_count=1  ovr_cals=on  ovr_actions=on  show_actions=on  action1_name=''  action1_cond=(None)  action2_name=''  action2_cond=(None)  action3_name=''  action3_cond=(None)  action4_name=''  action4_cond=(None)
  motohawk_fault_def9 : MotoHawk_lib/Fault Management Blocks/motohawk_fault_def  nam='Contactor_3_Fused'  mode=Disabled  id=['B1B58']  x=9  y=10  input_suspected=on  indeterminate=off  increment_xy=on  downsample_count=1  ovr_cals=on  ovr_actions=on  show_actions=on  action1_name=''  action1_cond=(None)  action2_name=''  action2_cond=(None)  action3_name=''  action3_cond=(None)  action4_name=''  action4_cond=(None)
  wires:
  In1/1 -> Bus Selector/1, Bus Selector1/1, Bus Selector2/1, Bus Selector4/1, Bus Selector5/1, Bus Selector7/1, Bus Selector8/1, Bus Selector11/1, Bus Selector10/1, Bus Selector9/1, Bus Selector6/1, Bus Selector3/1
  Bus Selector/1 -> Relational Operator/1  "<Contactor1>"
  [Contactor1] -> Relational Operator/2
  Relational Operator/1 -> motohawk_fault_def1/1
  Bus Selector1/1 -> Relational Operator1/1  "<Contactor1>"
  [Contactor1] -> Relational Operator1/2, Time Since Enabled (With Input)1/1
  Time Since Enabled (With Input)1/1 -> Relational Operator2/1
  motohawk_calibration/1 -> Relational Operator2/2
  Relational Operator1/1 -> Logical Operator/1
  Relational Operator2/1 -> Logical Operator/2
  Logical Operator/1 -> motohawk_fault_def2/1
  Bus Selector2/1 -> Relational Operator3/1  "<Contactor1>"
  [Contactor1] -> Relational Operator3/2
  Relational Operator3/1 -> motohawk_fault_def3/1
  Bus Selector3/1 -> Relational Operator4/1  "<Contactor2>"
  [Contactor2] -> Relational Operator4/2
  Relational Operator4/1 -> motohawk_fault_def4/1
  Bus Selector4/1 -> Relational Operator5/1  "<Contactor2>"
  [Contactor2] -> Relational Operator5/2, Time Since Enabled (With Input)2/1
  Time Since Enabled (With Input)2/1 -> Relational Operator6/1
  motohawk_calibration1/1 -> Relational Operator6/2
  Relational Operator5/1 -> Logical Operator1/1
  Relational Operator6/1 -> Logical Operator1/2
  Logical Operator1/1 -> motohawk_fault_def5/1
  Bus Selector5/1 -> Relational Operator7/1  "<Contactor2>"
  [Contactor2] -> Relational Operator7/2
  Relational Operator7/1 -> motohawk_fault_def6/1
  Bus Selector6/1 -> Relational Operator8/1  "<Contactor3>"
  [Contactor3] -> Relational Operator8/2
  Relational Operator8/1 -> motohawk_fault_def7/1
  Bus Selector7/1 -> Relational Operator9/1  "<Contactor3>"
  [Contactor3] -> Relational Operator9/2, Time Since Enabled (With Input)3/1
  Time Since Enabled (With Input)3/1 -> Relational Operator10/1
  motohawk_calibration2/1 -> Relational Operator10/2
  Relational Operator9/1 -> Logical Operator2/1
  Relational Operator10/1 -> Logical Operator2/2
  Logical Operator2/1 -> motohawk_fault_def8/1
  Bus Selector8/1 -> Relational Operator11/1  "<Contactor3>"
  [Contactor3] -> Relational Operator11/2
  Relational Operator11/1 -> motohawk_fault_def9/1
  Bus Selector9/1 -> Relational Operator12/1  "<Contactor4>"
  [Contactor4] -> Relational Operator12/2
  Relational Operator12/1 -> motohawk_fault_def10/1
  Bus Selector10/1 -> Relational Operator13/1  "<Contactor4>"
  [Contactor4] -> Relational Operator13/2, Time Since Enabled (With Input)4/1
  Time Since Enabled (With Input)4/1 -> Relational Operator14/1
  motohawk_calibration3/1 -> Relational Operator14/2
  Relational Operator13/1 -> Logical Operator3/1
  Relational Operator14/1 -> Logical Operator3/2
  Logical Operator3/1 -> motohawk_fault_def11/1
  Bus Selector11/1 -> Relational Operator15/1  "<Contactor4>"
  [Contactor4] -> Relational Operator15/2
  Relational Operator15/1 -> motohawk_fault_def12/1
